simulink model "simulation"  (R2019b)
settings: Solver=FixedStepAuto  StartTime=0.0  StopTime=10  FixedStep=0.01  MaxStep=100e-3  RelTol=1e-3
(part 2 of 2)

== stateflow chart simulation/Req12 ==
  note: The module responsible by test the requeriment twelve.
      |
      | Notice : i_ means input signals
      | 		o_ means output signals
      |
      | Input :
      | i_enable - Start the test. 1- Start test . 0 - Do nothing.
      | i_desiredTest - Test Number Value. All the modules recieve the
      | signal and decide either execute the test. Ex: Value "1" means that will being testing the requeriment 1.
      | i_IPCInd. 0 - Showing nothing ; 1 - Showing items .
      |
      |
      | Output :
      | o_TestResult - Result of test. 1 - Test ran correctly ; 2 - Test ran incorrectly.
      | o_TestDone - Test has been completed. 1 - Completed ;
      | o_keyfob - Signal that indicates if the key is inside or not from the car. 1 - Key inside ; 0 - Key outside.
      | o_keyCommand - Signal to lock or unlock the car. "1 - lock the car ; 0 - Unlock the car" ;  -1 - Do nothing.
      | o_doorCom - Signal to represent the opening the door. 1 - Opening ; 0 - Closing ; -1 - Do nothing.
  state state_ipcoff
    during :
    o_keyfobcom = 0;
    o_keyfob = 0;
    on after(200,msec):
    r_aux=1;
    exit:
    r_aux =0;
  state state_idle
    entry:
    r_aux=0;
  state state_ipcOn
    during :
    o_keyfobcom = 0;
    o_keyfob = 1;
    on after(500,msec):
    o_doorCom = 1;
    on after(1,sec):
    r_aux=1;
    exit:
    r_aux =0;
    o_doorCom = 0;
  state State_error
    during:
    o_TestResult =0;
    o_testDone =1 ;
    on after(300,msec):
    r_aux =1;
    exit :
    r_aux =0;
    o_keyfob = 0;
  state State_feat_ok
    entry :
    o_keyfob = 0;
    during:
    o_TestResult =1;
    o_testDone =1;
    on after(500,msec):
    r_aux =1;
    exit:
    r_aux =0;
    o_keyfob = 0;
  state state_update
    entry:
    r_aux = 0;
    during:
    on after(200,msec):
    o_TestResult =0;
    o_testDone = 0;
    r_aux =1 ;
    exit:
  (default) -> state_idle
  state_idle -> state_ipcoff : [i_enable==1 && i_desiredTest == 12 ]
  state_ipcoff -> State_error [order 2] : [r_aux==1 && i_IPCInd==1]
  state_update -> state_idle : [r_aux==1]
  state_ipcoff -> state_ipcOn [order 1] : [r_aux==1 && i_IPCInd==0]
  state_ipcOn -> State_error [order 2] : [r_aux==1 && i_IPCInd==0]
  state_ipcOn -> State_feat_ok [order 1] : [r_aux==1 && i_IPCInd==1]
  State_error -> state_update : [r_aux==1]
  State_feat_ok -> state_update : [r_aux==1]
  data: i_enable input; i_desiredTest input; o_TestResult output; o_testDone output; r_aux local; i_IPCInd input; o_keyfob output; o_keyfobcom output; o_doorCom output

== stateflow chart simulation/Req13 ==
  note: The module responsible by test the requeriment thirteen.
      |
      | Notice : i_ means input signals
      | 		o_ means output signals
      |
      | Input :
      | i_enable - Start the test. 1- Start test . 0 - Do nothing.
      | i_desiredTest - Test Number Value. All the modules recieve the
      | signal and decide either execute the test. Ex: Value "1" means that will being testing the requeriment 1.
      | i_ajarDoor. 1 - Door in aja state  ; 0 -  Door not in aja state .
      |
      |
      | Output :
      | o_TestResult - Result of test. 1 - Test ran correctly ; 0 - Test ran incorrectly.
      | o_TestDone - Test has been completed. 1 - Completed ;
      | o_keyCommand - Signal to lock or unlock the car. "1 - lock the car ; 0 - Unlock the car" ;  -1 - Do nothing.
      | o_doorajar. Signal to represent the opening the door. 1 - Opening ; 0 - Closing ; -1 - Do nothing.
  state state_testajarDoorTrue
    during:
    o_keyfobcommand = 0;
    o_doorAjar = 1;
    on after(200,msec):
    r_aux=1;
    exit:
    r_aux=0;
  state state_testajarDoorTrue1
    during:
    o_keyfobcommand = 0;
    o_doorAjar = 0;
    on after(500,msec):
    r_aux=1
    exit:
    r_aux=0;
  state state_idle
    entry:
    r_aux=0;
    o_doorAjar = 0;
    o_keyfobcommand = 0;
  state state_testCarlock
    during:
    o_keyfobcommand = 1;
    o_doorAjar = 1;
    on after(1,sec):
    r_aux=1
    exit:
    r_aux=0;
  state State_error
    during:
    o_TestResult =0;
    o_testDone =1 ;
    on after(100,msec):
    r_aux =1;
    exit :
    r_aux =0;
    o_doorAjar = 0;
  state State_feat_ok
    during:
    o_TestResult =1;
    o_testDone =1;
    on after(100,msec):
    r_aux =1;
    exit:
    r_aux =0;
  state state_update
    entry:
    r_aux = 0;
    on after(5,msec):
    during:
    o_TestResult =0;
    o_testDone = 0;
    r_aux =1 ;
    exit:
  state_testajarDoorTrue -> state_testajarDoorTrue1 [order 2] : [r_aux==1 && i_doorAjar == 1]
  state_testajarDoorTrue -> State_error [order 1] : [r_aux==1 && i_doorAjar == 0]
  (default) -> state_idle
  state_idle -> state_testajarDoorTrue : [i_enable==1 && i_desiredTest == 13 ]
  state_testajarDoorTrue1 -> State_error [order 2] : [r_aux==1 && i_doorAjar == 1]
  state_update -> state_idle : [r_aux==1]
  state_testajarDoorTrue1 -> state_testCarlock [order 1] : [r_aux==1 && i_doorAjar == 0]
  state_testCarlock -> State_error [order 2] : [r_aux==1 && i_doorAjar == 1]
  State_error -> state_update : [r_aux==1]
  state_testCarlock -> State_feat_ok [order 1] : [r_aux==1 && i_doorAjar == 0]
  State_feat_ok -> state_update : [r_aux==1]
  data: i_enable input; i_desiredTest input; i_doorAjar input; o_TestResult output; o_testDone output; r_aux local; o_doorAjar output int8; o_keyfobcommand output

== stateflow chart simulation/Req15 ==
  note: The module responsible by test the requeriment fifteen.
      |
      | Notice : i_ means input signals
      | 		o_ means output signals
      |
      | Input :
      | i_enable - Start the test. 1- Start test . 0 - Do nothing.
      | i_desiredTest - Test Number Value. All the modules recieve the
      | signal and decide either execute the test. Ex: Value "1" means that will being testing the requeriment 1.
      | i_gear -  geared State ; 1 - Park ; 0 - Engaged.
      | i_MotorStatus. 1 - On ; 0 - Off .
      |
      |
      | Output :
      |
      | o_TestResult - Result of test. 1 - Test ran correctly ; 0 - Test ran incorrectly.
      | o_TestDone - Test has been completed. 1 - Completed ;
      | o_keyComm - Signal to lock or unlock the car. "1 - lock the car ; 0 - Unlock the car" ;  -1 - Do nothing.
      | o_startButtom - Signal to start or off the car. 1- Car Start ; 0 - Car off.
      | o_keyfob - Signal that indicates if the key is inside or not from the car. 1 - Key inside ; 0 - Key outside.
      | o_gear = gear State ; 1 - Park ; 0 - Engaged.
  state state_gearParkOffCar
    entry:r_aux=0;
    during:
    o_keyfobcom = 0;
    on after(200,msec):
    o_keyfob =1;
    o_gear=1;
    on after(1,sec):
    o_startButtom =1;
    on after(2,sec):
    r_aux=1;
    exit :
    r_aux=0;
  state state_idle
    entry:
    r_aux=0;
  state State_error
    during:
    o_TestResult =0;
    o_testDone =1 ;
    on after(200,msec):
    r_aux =1;
    exit :
    r_aux =0;
  state state_gearParkOnCar
    entry:r_aux=0;
    during:
    o_keyfobcom = 0;
    on  after(200,msec):
    o_keyfob =1;
    o_gear=0;
    on after(400,msec):
    o_startButtom =0;
    on after(1,sec):
    r_aux=1;
    exit :
    r_aux=0;
  state state_update
    entry:
    r_aux = 0;
    on after(400,msec):
    during:
    o_TestResult =0;
    o_testDone = 0;
    r_aux =1 ;
    exit:
    o_keyfobcom = 0;
    o_keyfob =0;
    o_gear=0;
  state State_feat_ok
    during:
    o_TestResult =1;
    o_testDone =1;
    on after(200,msec):
    r_aux =1;
    exit:
    r_aux =0;
  state state_gear
    during :
    o_gear = 1;
    o_startButtom =0;
  (default) -> state_idle
  state_idle -> state_gearParkOffCar : [i_enable==1 && i_desiredTest == 15]
  state_gearParkOffCar -> state_gearParkOnCar [order 1] : [r_aux==1 && i_motorStatus==1 && i_gear ==1]
  state_gearParkOffCar -> State_error [order 2] : [(r_aux==1 && i_motorStatus==0) || (r_aux==1 && i_gear ~=1) ]
  state_update -> state_idle : [r_aux==1]
  state_gear -> State_error [order 2] : [after(500,msec) &&  i_motorStatus==1]
  state_gearParkOnCar -> State_error [order 2] : [r_aux==1 && i_motorStatus==0]
  State_error -> state_update : [r_aux==1]
  state_gearParkOnCar -> state_gear [order 1] : [r_aux==1 && i_motorStatus==1]
  state_gear -> State_feat_ok [order 1] : [after(500,msec)  && i_motorStatus==0]
  State_feat_ok -> state_update : [r_aux==1]
  data: i_enable input; i_desiredTest input; o_TestResult output; o_testDone output; r_aux local; i_motorStatus input; o_gear output; o_keyfob output; o_keyfobcom output; o_startButtom output; i_gear input

== stateflow chart simulation/Req16 ==
  state state_headLamp4 [commented out]
    entry:
    r_aux=0;
    during :
    o_levelluminosity = 1;
  state state_headLamp2 [commented out]
    entry:
    o_gear=1;
    o_keyfob = 1;
    o_headLamp = 2 ;
  state state_headLamp3 [commented out]
    entry:
    o_headLamp = 3 ;
  state state_idle [commented out]
    entry:
    r_aux=0;
    o_keyfob = 0 ;
  state state_headLamp5 [commented out]
    entry:
    r_aux=0;
    during :
    o_levelluminosity = 2;
  note: The module responsible by test the requeriment sixteen.
      |
      | Notice : i_ means input signals
      | 		o_ means output signals
      |
      | Input :
      | i_enable - Start the test. 1- Start test . 0 - Do nothing.
      | i_desiredTest - Test Number Value. All the modules recieve the
      | signal and decide either execute the test. Ex: Value "1" means that will being testing the requeriment 1.
      | i_MotorStatus. 1 - On ; 0 - Off .
      | i_headLampLowBeam. 1 - Lamp  On ; 0 - Lamp Off.
      | i_headLampPark. 1 - Lamp On ; 0 - Lamp Off.
      | i_headLampHigh. 1 - Lamp On ; 0 - Lamp Off.
      |
      |
      | Output :
      | o_TestResult - Result of test. 1 - Test ran correctly ; 2 - Test ran incorrectly.
      | o_TestDone - Test has been completed. 1 - Completed ;
      | o_keyfobComm - Signal to lock or unlock the car. "1 - lock the car ; 0 - Unlock the car" ;  -1 - Do nothing.
      | o_startButtom - Signal to start or off the car. 1- Car Start ; 0 - Car Off.
      | o_keyfob - Signal that indicates if the key is inside or not from the car. 1 - Key inside ; 0 - Key outside.
      | o_levelluminosity - Luminosity Level. Range 0 ~ 4.
  state State_error [commented out]
    during:
    o_TestResult =0;
    o_testDone =1 ;
    on after(200,msec):
    r_aux =1;
    exit :
    r_aux =0;
  state state_headLamp6 [commented out]
    entry:
    o_levelluminosity = 4;
  state state_update [commented out]
    entry:
    r_aux = 0;
    on after(200,msec):
    during:
    o_TestResult =0;
    o_testDone = 0;
    r_aux =1 ;
    exit:
    o_keyfob = 0;
    o_keyfobCom = 0;
    o_headLamp=0;
    o_startButtom = 0;
  state State_feat_ok [commented out]
    during:
    o_TestResult =1;
    o_testDone =1;
    on after(200,msec):
    r_aux =1;
    exit:
    r_aux =0;
  state state_headLamp1 [commented out]
    entry: r_aux=0;
    during:
    o_keyfob = 1;
    o_keyfobCom = 0 ;
    on after(200,msec):
    o_startButtom =1;
    on after(400,msec):
    o_headLamp=0;
    on after(600,msec):
    o_startButtom =0;
    r_aux=1;
    exit:
    r_aux = 0;
  state StateTurnOnCar
    during :
    o_keyfobCom = 0;
    on after(50,msec):
    o_keyfob = 1;
    on after(100,msec):
    o_gear = 1;
    o_headLamp = 0;
    on after(150,msec):
    o_startButtom = 1;
  state state_tryTurnDown_Car
    during :
    o_startButtom = 0;
  state state_tryTurnDown_Car2
    during :
    o_headLamp = 0;
  state stateTurnOnHeadLamp
    during :
    o_headLamp = 1;
  state state_idle1
    entry:
    r_aux=0;
    o_keyfob = 0 ;
    o_levelluminosity = 4;
  state State_error1
    during:
    o_TestResult =0;
    o_testDone =1 ;
    on after(200,msec):
    r_aux =1;
    exit :
    r_aux =0;
  state state_update1
    entry:
    r_aux = 0;
    on after(200,msec):
    during:
    o_TestResult =0;
    o_testDone = 0;
    r_aux =1 ;
    exit:
    o_keyfob = 0;
    o_keyfobCom = 0;
    o_headLamp=0;
    o_startButtom = 0;
  state State_feat_ok1
    during:
    o_TestResult =1;
    o_testDone =1;
    on after(200,msec):
    r_aux =1;
    exit:
    r_aux =0;
  (default) -> state_idle [commented out]
  state_headLamp4 -> state_headLamp5 [commented out] : [after(500,msec)  && i_headLampPark==0 && i_headLampLowBeam ==1]
  state_headLamp3 -> state_headLamp4 [commented out] : [after(500,msec)]
  state_update -> state_idle [commented out] : [r_aux==1]
  state_headLamp2 -> state_headLamp3 [commented out] : [after(500,msec) && i_headLampPark ==0 && i_headLampLowBeam ==1 ]
  state_idle -> state_headLamp2 [commented out] : [i_enable==1 && i_desiredTest ==16]
  state_headLamp4 -> State_error [commented out] : [after(25,sec) &&(i_headLampPark ~=0 || i_headLampLowBeam ~=0 )]
  state_headLamp2 -> State_error [commented out] : [after(500,sec) &&(i_headLampPark ~=0 || i_headLampLowBeam ~=1 )]
  state_headLamp5 -> State_error [commented out] : [after(25,sec)  && ( i_headLampPark ~=1 || i_headLampLowBeam ~=0)]
  state_headLamp5 -> state_headLamp6 [commented out] : [after(500,msec) && i_headLampPark==1 && i_headLampLowBeam ==0]
  state_headLamp6 -> State_error [commented out] : [after(25,sec)  && (i_headLampPark~=0 || i_headLampLowBeam ~=0)]
  state_headLamp1 -> State_error [commented out] : [(r_aux==1 && i_motorStatus==1) || (r_aux ==1  && i_headLampPark~=0 || i_headLampLowBeam ~=0) ]
  State_error -> state_update [commented out] : [r_aux==1]
  State_feat_ok -> state_update [commented out] : [r_aux==1]
  state_headLamp6 -> state_headLamp1 [commented out] : [after(25,sec) && i_headLampHigh ==0 && i_headLampPark==0 && i_headLampLowBeam ==0]
  state_headLamp1 -> State_feat_ok [commented out] : [r_aux==1 && i_motorStatus==0 && i_headLampPark==0 && i_headLampLowBeam ==0 ]
  (default) -> state_idle1
  state_tryTurnDown_Car -> state_tryTurnDown_Car2 [order 2] : [after(1,sec) && i_motorStatus ==1]
  StateTurnOnCar -> stateTurnOnHeadLamp [order 2] : [after(300,msec) && i_motorStatus==1]
  stateTurnOnHeadLamp -> state_tryTurnDown_Car [order 1] : [after(100,msec) && i_headLampPark == 1 && i_headLampLowBeam == 0 ]
  state_update1 -> state_idle1 : [r_aux==1]
  state_idle1 -> StateTurnOnCar : [i_enable==1 && i_desiredTest ==16]
  stateTurnOnHeadLamp -> State_error1 [order 2] : [after(100,msec) && i_headLampPark ~= 1 && i_headLampLowBeam ~= 0 ]
  state_tryTurnDown_Car2 -> State_error1 [order 2] : [after(500,msec) && i_motorStatus ==1]
  state_tryTurnDown_Car2 -> State_feat_ok1 [order 1] : [after(500,msec) && i_motorStatus ==0]
  state_tryTurnDown_Car -> State_error1 [order 1] : [after(1,sec) && i_motorStatus ==0]
  StateTurnOnCar -> State_error1 [order 1] : [after(300,msec) && i_motorStatus==0]
  State_error1 -> state_update1 : [r_aux==1]
  State_feat_ok1 -> state_update1 : [r_aux==1]
  data: i_enable input; i_desiredTest input; o_TestResult output; o_testDone output; r_aux local; o_keyfobCom output; o_startButtom output; o_keyfob output; o_headLamp output; i_motorStatus input; i_headLampPark input; i_headLampLowBeam input; i_headLampHigh input; o_levelluminosity output double; o_gear output

== stateflow chart simulation/Req17 ==
  note: The module responsible by test the requeriment seventeen.
      |
      | Notice : i_ means input signals
      | 		o_ means output signals
      |
      | Input :
      | i_enable - Start the test. 1- Start test . 0 - Do nothing.
      | i_desiredTest - Test Number Value. All the modules recieve the
      | signal and decide either execute the test. Ex: Value "1" means that will being testing the requeriment 1.
      | i_lampValue. 1- Turn Lamp On ; 0 - Turn Lamp Off .
      |
      |
      | Output :
      | o_TestResult - Result of test. 1 - Test ran correctly ; 2 - Test ran incorrectly.
      | o_TestDone - Test has been completed. 1 - Completed ;
      | o_keyfobComm - Signal to lock or unlock the car. "1 - lock the car ; 0 - Unlock the car" ;  -1 - Do nothing.
      | o_keyfob - Signal that indicates if the key is inside or not from the car. 1 - Key inside ; 0 - Key outside.
  state state_testBlinkUnlockTheCar
    entry: r_aux = 0;
    during :
    on after(5,sec):
    o_keyfobcom = 0;
    on after(5.1,sec):
    if (i_lamp_value ~=r_lamp_value )
    r_blink = r_blink +1;
    r_lamp_value = i_lamp_value ;
    end
    exit:
    r_blink  = 0;
  state state_idle
    entry:
    r_aux=0;
    r_lamp_value = i_lamp_value ;
    o_ketfob = 0;
    o_keyfobcom = 1;
    r_blink = 0;
  state state_testBlinkUnlockTheCar1
    entry: r_aux = 0;
    r_lamp_value = i_lamp_value;
    during :
    o_keyfobcom = 1;
    if (i_lamp_value ~=r_lamp_value )
    r_blink = r_blink +1;
    r_lamp_value = i_lamp_value ;
    end
  state State_feat_ok
    during:
    o_TestResult =1;
    o_testDone =1;
    on after(200,msec):
    r_aux =1;
    exit:
    r_aux =0;
  state State_error
    during:
    o_TestResult =0;
    o_testDone =1 ;
    on after(200,msec):
    r_aux =1;
    exit :
    r_aux =0;
  state state_update
    entry:
    r_aux = 0;
    on after(500,msec):
    during:
    o_TestResult =0;
    o_testDone = 0;
    r_aux =1 ;
    exit:
    o_keyfobcom = 0;
  (default) -> state_idle
  state_idle -> state_testBlinkUnlockTheCar : [i_enable==1 && i_desiredTest ==17  ]
  state_testBlinkUnlockTheCar -> state_testBlinkUnlockTheCar1 [order 1] : [after(30,sec) && r_blink==2]
  state_update -> state_idle : [r_aux==1]
  state_testBlinkUnlockTheCar -> State_error [order 2] : [after(26,sec) && r_blink~=2]
  state_testBlinkUnlockTheCar1 -> State_error [order 2] : [after(40,sec) && r_blink~=4]
  state_testBlinkUnlockTheCar1 -> State_feat_ok [order 1] : [after(40,sec) && r_blink==4]
  State_feat_ok -> state_update : [r_aux==1]
  State_error -> state_update : [r_aux==1]
  data: i_enable input int8; i_desiredTest input int8; o_TestResult output int8; o_testDone output int8; r_aux local; r_blink local; r_lamp_value local; i_lamp_value input int8; o_ketfob output int8; o_keyfobcom output int8

== stateflow chart simulation/Req18 ==
  note: The module responsible by test the requeriment nineteen.
      |
      | Notice : i_ means input signals
      | 		o_ means output signals
      |
      | Input :
      | i_enable - Start the test. 1- Start test . 0 - Do nothing.
      | i_desiredTest - Test Number Value. All the modules recieve the
      | signal and decide either execute the test. Ex: Value "1" means that will being testing the requeriment 1.
      | i_DRL. 1- DRL  Lamp On ; 0 - DRL Lamp Off .
      |
      |
      | Output :
      | o_TestResult - Result of test. 1 - Test ran correctly ; 2 - Test ran incorrectly.
      | o_TestDone - Test has been completed. 1 - Completed ;
      | o_keyfobComm - Signal to lock or unlock the car. "1 - lock the car ; 0 - Unlock the car" ;  -1 - Do nothing.
  state state_DrlOn
    entry :
    r_aux=0;
    during :
    on after(20,sec):
    o_keyfobcom = 0;
    on after(40,sec):
    r_aux = 1 ;
    exit :
    r_aux = 0;
  state state_DrlOff
    entry : r_aux=0;
    during :
    o_keyfobcom =1;
    on after(40,sec):
    r_aux = 1 ;
    exit :
    r_aux = 0 ;
  state state_idle
    entry:
    r_aux=0;
    o_keyfobcom = 1;
  state State_feat_ok
    during:
    o_TestResult =1;
    o_testDone =1;
    on after(200,msec):
    r_aux =1;
    exit:
    r_aux =0;
  state State_error
    during:
    o_TestResult =0;
    o_testDone =1 ;
    on after(200,msec):
    r_aux =1;
    exit :
    r_aux =0;
  state state_update
    entry:
    r_aux = 0;
    on after(300,msec):
    during:
    o_TestResult =-1;
    o_testDone = 0;
    r_aux =1 ;
    exit:
  (default) -> state_idle
  state_idle -> state_DrlOn : [i_enable==1 && i_desiredTest == 18 ]
  state_DrlOn -> state_DrlOff [order 1] : [r_aux==1 && i_DRL==1]
  state_DrlOn -> State_error [order 2] : [r_aux==1 && i_DRL==0]
  state_DrlOff -> State_error [order 2] : [r_aux==1 && i_DRL==1]
  state_DrlOff -> State_feat_ok [order 1] : [r_aux==1 && i_DRL==0]
  state_update -> state_idle : [r_aux==1]
  State_feat_ok -> state_update : [r_aux==1]
  State_error -> state_update : [r_aux==1]
  data: i_enable input int8; i_desiredTest input; o_TestResult output; o_testDone output; i_DRL input; r_aux local double; o_keyfobcom output

== stateflow chart simulation/"Req 2" ==
  note: The module responsible by test the requeriment one.
      |
      | Notice : i_ means input signals
      | 		o_ means output signals
      |
      | Input :
      | i_enable - Start the test. 1- Start test . 0 - Do nothing.
      | i_desiredTest - Test Number Value. All the modules recieve the
      | signal and decide either execute the test. Ex: Value "1" means that will being testing the requeriment 1.
      | i_WindowRightState = Windows State. 1- Windows Opening  ; 0 - Windows Closing ;  -1 - Do nothing.
      | i_WindowLeftState = Windows State. 1- Windows Opening  ; 0 - Windows Closing ;  -1 - Do nothing.
      | Output :
      | o_keyfob - Signal that indicates if the key is inside or not from the car. 1 - Key inside ; 0 - Key outside.
      | o_startButtom - Signal to start or off the car. 1- Car Start ; 0 - Car off.
      | o_WindowValue - Signal to move the windows " 1 - Opening ; 0- Closing ; -1 - Do Nothing  ;
      | o_gear = gear State ; 1 - Park ; 0 - Engaged.
      | o_keyfobCommand - Signal to lock or unlock the car. "1 - lock the car ; 0 - Unlock the car" ;  -1 - Do nothing.
      | o_TestResult - Result of test. 1 - Test ran correctly ; 2 - Test ran incorrectly.
      | o_TestDone - Test has been completed. 1 - Completed ;
  state State_idle
    entry :
    r_aux=0;
    r_count = 1 ;
    r_error = 0;
    o_startButtom = 0;
    o_keyfobCommand = 0;
    o_gear = 0 ;
    o_keyfob=0;
    o_WindowValue = -1;
  state state_readyingSystem
    during:
    o_keyfob =1;
    o_keyfobCommand = 0 ;
    o_gear = 1 ;
    on after(0.5,sec):
    o_startButtom = 1;
    on after(1.5,sec):
    r_aux=1;
    exit :
    r_aux=0;
  state state_testCarOn
    during:
    o_WindowValue =0 ;
    on after(2,sec):
    r_aux=1;
    exit :
    r_aux=0;
  state state_testCarOff
    during:
    o_startButtom = 0;
    %on after(300,msec):
    %o_keyfob =0;
    %on after(500,msec):
    %o_keyfobCommand = 1 ;
    on after(2,sec):
    o_WindowValue= 0;
    on after(3,sec):
    r_aux=1;
    exit :
    r_aux=0;
    o_WindowValue= -1;
  state State_error
    during:
    o_TestResult =0;
    o_testDone =1 ;
    on after(200,msec):
    r_aux =1;
    exit :
    r_aux =0;
  state state_temp
  state state_testAfter10sec
    entry:
    o_WindowValue= 0;
  state state_update
    entry:
    r_aux = 0;
    during:
    o_TestResult =0;
    o_testDone = 0;
    on after(500,msec):
    r_aux =1 ;
    exit:
  state State_feat_ok
    during:
    o_TestResult =1;
    o_testDone =1;
    on after(200,msec):
    r_aux =1;
    exit:
    r_aux =0;
  (default) -> State_idle
  State_idle -> state_readyingSystem : [i_enable==1 && i_desiredTest ==2 ]
  state_readyingSystem -> state_testCarOn : [r_aux==1]
  state_testCarOn -> state_testCarOff [order 2] : [(i_WindowRightState==0 && i_WindowLeftState == 0)  && r_aux==1]
  state_update -> State_idle : [r_aux==1]
  state_testCarOn -> State_error [order 1] : [(i_WindowRightState~=0 || i_WindowLeftState ~= 0)   && r_aux==1]
  state_testCarOff -> State_error [order 2] : [(i_WindowRightState~=0 || i_WindowLeftState ~= 0)   && r_aux==1]
  state_testAfter10sec -> State_error [order 1] : [(i_WindowRightState~=-1 && i_WindowLeftState ~= -1) && after(300,msec)]
  State_error -> state_update : [r_aux==1]
  state_testCarOff -> state_temp [order 1] : [(i_WindowRightState==0 && i_WindowLeftState == 0)  && r_aux==1]
  state_temp -> state_testAfter10sec : [after(11,sec)]
  state_testAfter10sec -> State_feat_ok [order 2] : [(i_WindowRightState==-1 && i_WindowLeftState == -1) && after(300,msec)]
  State_feat_ok -> state_update : [r_aux==1]
  data: o_TestResult output; r_aux local; i_desiredTest input; i_enable input; r_error local; o_testDone output; r_count local; o_keyfob output; i_WindowRightState input; o_keyfobCommand output; o_startButtom output; o_WindowValue output; o_gear output; i_WindowLeftState input

== stateflow chart simulation/Req 4 ==
  state state_test_unlock_doors [commented out]
    during:
    o_keyfob =1;
    o_keyfobCom = 0;
    on after(10,msec):
    o_lockDoor = 0 ;
    on after(1.5,sec):
    r_aux = 1;
    exit : r_aux = 0;
  note: The module responsible by test the requeriment four.
      |
      | Notice : i_ means input signals
      | 		o_ means output signals
      |
      | Input :
      | i_enable - Start the test. 1- Start test . 0 - Do nothing.
      | i_desiredTest - Test Number Value. All the modules recieve the
      | signal and decide either execute the test. Ex: Value "1" means that will being testing the requeriment 1.
      | i_WindowsStateAnd - And condition with the WindowState . 1-  Both is Windows Closing ; 0 - Windows Opening ;  -1 - Do nothing.
      | i_WindowsStateAnd - And condition with the DoorState. 1 - Both Door are closing  ;  0 - Some Door is opening ;  -1 Do nothing.
      | i_WindowsStateOr - Or condition with the DoorState. 1 - Some Door is closing ;  0 - Both Door are opening ;  -1 Do nothing.
      | i_stateDoorAnd - And condition with the Door Lock State. 1 - Both Door are Locked; 0 - Some Door is unlocked; -1 Do nothing.
      | i_stateDoorOR - Or condition with the Door Lock State. 1 - Some Door is locked;  0 - Both Door are unlocked ;  -1 Do nothing.
      |
      | Output :
      | o_TestResult - Result of test. 1 - Test ran correctly ; 2 - Test ran incorrectly.
      | o_TestDone - Test has been completed. 1 - Completed .
      | o_keyfob - Signal that indicates if the key is inside or not from the car. 1 - Key inside ; 0 - Key outside.
      | o_keyfobComm - Signal to lock or unlock the car. "1 - lock the car ; 0 - Unlock the car" ;  -1 - Do nothing.
      | o_WindowState - Signal to move the windows " 0 - Opening ; 1- Closing ; -1 - Do Nothing  ;
      | o_lockDoor = Lock Door ; 1 - Lock the doors; 0 - unlock the doors.
  state State_idle
    entry :
    r_aux=0;
    o_TestResult = 0;
    o_lockDoor=-1;
    during:
  state state_test_lock_doors
    during:
    o_keyfob =1;
    o_keyfobCom = 0;
    on after(200,msec):
    o_lockDoor = 1 ;
    on after(300,msec):
    o_gear =1;
    on after(400,msec):
    o_startButtom =1 ;
    on after(1.7,sec):
    r_aux = 1;
    exit : r_aux = 0;
  state state_test_windowsTest
    during:
    o_keyfob =1;
    o_keyfobCom = 0;
    on after(100,msec):
    o_startButtom =1 ;
    on after(600,msec):
    o_DDSCommand = 0;
    on after(1,sec):
    o_windowState = 0 ;
    on after(2.5,sec):
    r_aux = 1;
    exit : r_aux = 0;
  state State_error
    during:
    o_TestResult =0;
    o_testDone =1 ;
    on after(100,msec):
    r_aux =1;
    exit :
    r_aux =0;
  state state_WindowsTest1
    during:
    o_keyfob =1;
    o_keyfobCom = 0;
    on after(100,msec):
    o_startButtom =1 ;
    on after(800,msec):
    o_DDSCommand = 1;
    on after(2.4,sec):
    o_windowState = 1 ;
    on after(4,sec):
    r_aux = 1;
    exit : r_aux = 0;
  state State_feat_ok
    entry :
    o_lockDoor=0;
    o_keyfob = 0 ;
    o_keyfobCom =0;
    during:
    o_TestResult =1;
    o_testDone =1;
    on after(500,msec):
    r_aux =1;
    exit:
    r_aux =0;
  state state_update
    entry:
    o_lockDoor=0;
    o_keyfob = 0 ;
    o_keyfobCom =0;
    r_aux = 0;
    on after(500,msec):
    during:
    o_TestResult =0;
    o_testDone = 0;
  (default) -> ? [commented out] : [r_aux ==1 &&  i_stateDoorRight==0 && i_stateDoorLeft ==0]
  state_test_unlock_doors -> ? [commented out] : [r_aux ==1 &&  i_stateDoorRight ~=0 && i_stateDoorLeft ~=0]
  (default) -> State_idle
  State_idle -> state_test_lock_doors : [i_enable==1 && i_desiredTest ==4 ]
  state_test_lock_doors -> state_test_windowsTest [order 1] : [r_aux ==1 &&  i_stateDoorRight==1 && i_stateDoorLeft ==1]
  state_update -> State_idle : [after(100,msec)]
  state_test_windowsTest -> State_error [order 2] : [r_aux ==1 &&  i_windowStateLeft~=-1 && i_windowStateRight~=-1]
  state_test_lock_doors -> State_error [order 2] : [r_aux ==1 &&  i_stateDoorRight~=1 && i_stateDoorLeft ~=1]
  state_test_windowsTest -> state_WindowsTest1 [order 1] : [r_aux ==1 &&  i_windowStateLeft==-1 && i_windowStateRight==-1]
  state_WindowsTest1 -> State_error [order 2] : [r_aux ==1 &&  i_windowStateLeft~=1 && i_windowStateRight~=1]
  State_error -> state_update : [r_aux==1]
  state_WindowsTest1 -> State_feat_ok [order 1] : [r_aux ==1 &&  i_windowStateLeft==1 && i_windowStateRight==1]
  State_feat_ok -> state_update : [r_aux==1]
  data: o_TestResult output; r_aux local; i_desiredTest input; i_enable input; o_testDone output; i_stateDoorRight input; i_stateDoorLeft input; o_keyfob output; o_keyfobCom output; o_lockDoor output; o_windowState output; i_windowStateLeft input; o_startButtom output; o_DDSCommand output; i_windowStateRight input; o_gear output
